simulink model "M182_Lab1"  (R2019b)
settings: Solver=VariableStepAuto  StartTime=0.0  StopTime=20  RelTol=1e-3
settings Model: Creator=scjcb  LastModifiedBy=scjcb

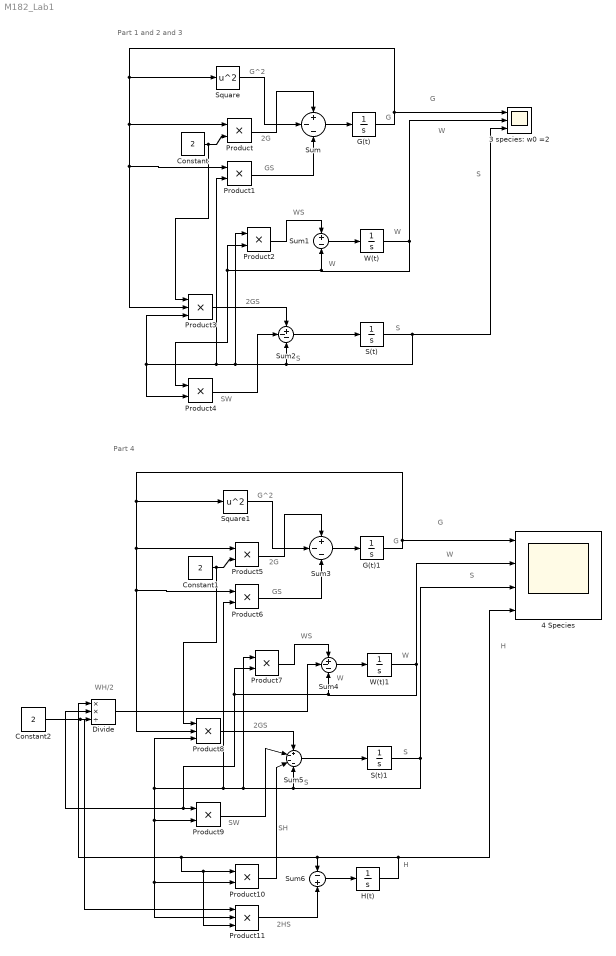
== system M182_Lab1 ==
  note: H
  note: H
  note: 2HS
  note: SH
  note: WH/2
  note: S
  note: Part 1 and 2 and 3
  note: W
  note: G
  note: 2GS
  note: SW
  note: S
  note: S
  note: W
  note: WS
  note: W
  note: GS
  note: 2G
  note: G^2
  note: G
  note: Part 4
  note: SW
  note: S
  note: W
  note: W
  note: 2G
  note: S
  note: WS
  note: G^2
  note: G
  note: S
  note: 2GS
  note: G
  note: W
  note: GS
  3 species: w0 =2 : Scope  NumInputPorts=3
  4 Species : Scope  NumInputPorts=4
  Constant : Constant  Value=2
  Constant1 : Constant  Value=2
  Constant2 : Constant  Value=2
  Divide : Product  Inputs=**/
  G(t) : Integrator  InitialCondition=2
  G(t)1 : Integrator  InitialCondition=2
  H(t) : Integrator  InitialCondition=2
  Product{,1..2,4..7,9..10} (9 alike) : Product
  Product11 : Product  Inputs=3
  Product3 : Product  Inputs=3
  Product8 : Product  Inputs=3
  S(t) : Integrator  InitialCondition=2
  S(t)1 : Integrator  InitialCondition=2
  Square : Math  Operator=square  SignedPower=off  SaturateOnIntegerOverflow=on
  Square1 : Math  Operator=square  SignedPower=off  SaturateOnIntegerOverflow=on
  Sum{,2..4} (4 alike) : Sum  Inputs=+--
  Sum1 : Sum  Inputs=+-
  Sum5 : Sum  Inputs=+---
  Sum6 : Sum  Inputs=-+
  W(t) : Integrator  InitialCondition=2
  W(t)1 : Integrator  InitialCondition=2
  wires:
  G(t)/1 -> Product1/1, Product3/2, Product/1, Square/1, 3 species: w0 =2/1
  Constant/1 -> Product3/1, Product/2
  Product/1 -> Sum/1
  Square/1 -> Sum/2
  Product1/1 -> Sum/3
  Sum/1 -> G(t)/1
  W(t)/1 -> Sum1/2, Product4/1, Product2/2, 3 species: w0 =2/2
  Product2/1 -> Sum1/1
  S(t)/1 -> Product2/1, Product1/2, Product4/2, Product3/3, Sum2/3, 3 species: w0 =2/3
  Product3/1 -> Sum2/1
  Sum2/1 -> S(t)/1
  Sum1/1 -> W(t)/1
  Product4/1 -> Sum2/2
  Product7/1 -> Sum4/1
  Product8/1 -> Sum5/1
  Constant1/1 -> Product8/1, Product5/2
  Sum4/1 -> W(t)1/1
  S(t)1/1 -> Sum5/4, Product7/1, Product6/2, Product11/2, Product10/2, Product9/2, Product8/3, 4 Species/3
  Sum5/1 -> S(t)1/1
  Square1/1 -> Sum3/2
  W(t)1/1 -> Sum4/3, Divide/2, Product9/1, Product7/2, 4 Species/2
  Product9/1 -> Sum5/2
  G(t)1/1 -> Product6/1, Product8/2, Product5/1, Square1/1, 4 Species/1
  Product5/1 -> Sum3/1
  Product6/1 -> Sum3/3
  Sum3/1 -> G(t)1/1
  Constant2/1 -> Product11/1, Divide/3
  H(t)/1 -> 4 Species/4, Sum6/1, Product11/3, Product10/1, Divide/1
  Divide/1 -> Sum4/2
  Product10/1 -> Sum5/3
  Product11/1 -> Sum6/2
  Sum6/1 -> H(t)/1
